simulink model "sim2_2_3"  (R2021a)
settings: Solver=VariableStepAuto  StartTime=0.0  StopTime=1  RelTol=1e-3
libraries: simulink x2
settings Model: Creator=zhaitia4  LastModifiedBy=zhaitia4

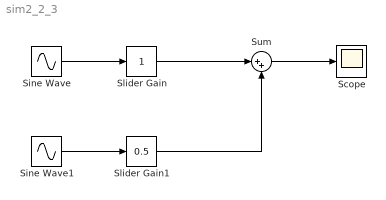
== system sim2_2_3 ==
  Scope : Scope
  Sine Wave : Sin  Frequency=2 * pi* 1000  SampleTime=1/48000  VectorParams1D=off
  Sine Wave1 : Sin  Frequency=2 * pi* 2000  SampleTime=1/48000  VectorParams1D=off
  Slider Gain : simulink/Math Operations/Slider Gain  gain=1  low=0  high=2
  Slider Gain1 : simulink/Math Operations/Slider Gain  gain=0.5  low=0  high=1
  Sum : Sum  Inputs=|++
  wires:
  Sine Wave1/1 -> Slider Gain1/1
  Sine Wave/1 -> Slider Gain/1
  Slider Gain/1 -> Sum/1
  Slider Gain1/1 -> Sum/2
  Sum/1 -> Scope/1
